simulink model "dentrosis"  (R2024b)
settings: Solver=ode45  StartTime=0.0  StopTime=10.0  MaxStep=1e-3  RelTol=1e-3
libraries: slpidlib x1
settings Model: Creator=Dell
settings DataIOCC: ReturnWorkspaceOutputs=off  TimeSaveName=t
settings DebuggingCC: AlgebraicLoopMsg=none  ArtificialAlgebraicLoopMsg=none  InheritedTsInSrcMsg=none
settings RTWCC: GPUComputeCapability=3.5

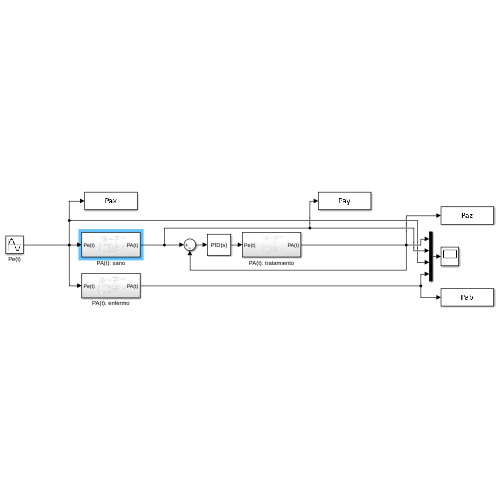
[thumbnail: Simulink's stored preview of the top-level diagram]
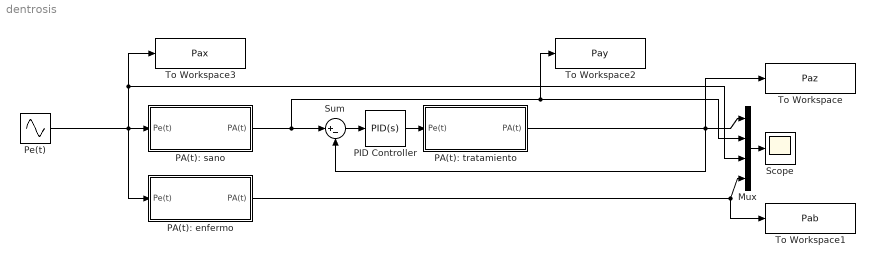
== system dentrosis ==
  Mux : Mux
  PA(t): enfermo : Subsystem
  PA(t): sano : Subsystem
  PA(t): tratamiento : Subsystem
  PID Controller : slpidlib/PID Controller  Controller=PID  Form=Parallel  TimeDomain=Continuous-time  UseExternalTs=off  SampleTime=-1  IntegratorMethod=Forward Euler  FilterMethod=Forward Euler  ControllerParametersSource=internal  P=7504.3128  I=40028.7836  UseKiTs=off  D=312.5866  UseExternalDerivativeSource=off  N=104491.5556  UseFilter=on  TunerSelectOption=Transfer Function Based (PID Tuner App)  InitialConditionSource=internal  InitialConditionForIntegrator=0  InitialConditionForFilter=0  DifferentiatorICPrevScaledInput=0  ExternalReset=none  TrackingMode=off  Kt=1  LimitOutput=off  SatLimitsSource=internal  UpperSaturationLimit=inf  LowerSaturationLimit=-inf  LinearizeAsGain=on  AntiWindupMode=none  Kb=1  LimitIntegrator=off  UpperIntegratorSaturationLimit=inf  LowerIntegratorSaturationLimit=-inf  POutMin=[]  POutMax=[]  IOutMin=[]  IOutMax=[]  DOutMin=[]  DOutMax=[]  NOutMin=[]  NOutMax=[]  SumOutMin=[]  SumOutMax=[]  SaturationOutMin=[]  SaturationOutMax=[]  PParamMin=[]  PParamMax=[]  IParamMin=[]  IParamMax=[]  DParamMin=[]  DParamMax=[]  NParamMin=[]  NParamMax=[]  KbParamMin=[]  KbParamMax=[]  KtParamMin=[]  KtParamMax=[]  KbOutMin=[]  KbOutMax=[]  KtOutMin=[]  KtOutMax=[]  IntegratorOutMin=[]  IntegratorOutMax=[]  FilterOutMin=[]  FilterOutMax=[]  SumI1OutMin=[]  SumI1OutMax=[]  SumI2OutMin=[]  SumI2OutMax=[]  SumI3OutMin=[]  SumI3OutMax=[]  SumI4OutMin=[]  SumI4OutMax=[]  SumDOutMin=[]  SumDOutMax=[]  DifferentiatorOutMin=[]  DifferentiatorOutMax=[]  FilterDiffOutCoefMin=[]  FilterDiffOutCoefMax=[]  ReciprocalOutMin=[]  ReciprocalOutMax=[]  SumDenOutMin=[]  SumDenOutMax=[]  SumNumOutMin=[]  SumNumOutMax=[]  DivideOutMin=[]  DivideOutMax=[]  UdiffTsProdOutMin=[]  UdiffTsProdOutMax=[]  NTsProdOutMin=[]  NTsProdOutMax=[]  UintegralTsProdOutMin=[]  UintegralTsProdOutMax=[]  UngainTsProdOutMin=[]  UngainTsProdOutMax=[]  ClampingZeroOutDataTypeStr=Inherit: Inherit via back propagation  ClampingZeroOutMin=[]  ClampingZeroOutMax=[]  FilterDenConstantOutDataTypeStr=Inherit: Inherit via back propagation  FilterDenConstantOutMin=[]  FilterDenConstantOutMax=[]  PCopyOutDataTypeStr=Inherit: Inherit via back propagation  PCopyOutMin=[]  PCopyOutMax=[]  NCopyOutDataTypeStr=Inherit: Inherit via back propagation  NCopyOutMin=[]  NCopyOutMax=[]  IntegratorContinuousStateAttributes=''  IntegratorStateMustResolveToSignalObject=off  IntegratorRTWStateStorageClass=Auto  FilterContinuousStateAttributes=''  FilterStateMustResolveToSignalObject=off  FilterRTWStateStorageClass=Auto  ParallelPVariant=InternalParameters  IdealPVariant=Disabled  IVariant=InternalParameters  DVariant=InternalParameters  IntegratorVariant=Continuous  SatVariant=Disabled  AWVariant=Passthrough  PCopyVariant=Disabled  TRVariant=Disabled  FdbkBlocksVariant=Forward  IdealPFdbkVariant=Disabled  SatFdbkVariant=Disabled  DerivativeFilterVariant=ContFilter  NVariant=InternalParameters  NCopyVariant=Disabled  FilterICVariant=InternalICsFilter  IntegratorICVariant=InternalICs  ExternalResetVariant=Disabled  TRSumVariant=Passthrough  SumFdbkVariant=Disabled  SumVariant=Sum_PID  TsampFilterVariant=InternalTs  TsampNgainVariant=Passthrough  TsampIntegralVariant=Disabled_SignalSpec  ExternalSaturationOutDataTypeStr=Inherit: Same as second input  DerivativeSourceVariant=ErrorSignal  PreIntVariant=InternalPreInt
  Pe(t) : Sin  Frequency=1.5
  Scope : Scope
  Sum : Sum  Inputs=|+-
  To Workspace : ToWorkspace  VariableName=Paz  SampleTime=-1
  To Workspace1 : ToWorkspace  VariableName=Pab  SampleTime=-1
  To Workspace2 : ToWorkspace  VariableName=Pay  SampleTime=-1
  To Workspace3 : ToWorkspace  VariableName=Pax  SampleTime=-1
  wires:
  Mux/1 -> Scope/1
  Sum/1 -> PID Controller/1
  PID Controller/1 -> PA(t): tratamiento/1(Pe(t))
  PA(t): tratamiento/1(PA(t)) -> To Workspace/1, Mux/1, Sum/2
  PA(t): sano/1(PA(t)) -> To Workspace2/1, Mux/2, Sum/1
  Pe(t)/1 -> PA(t): enfermo/1(Pe(t)), PA(t): sano/1(Pe(t)), To Workspace3/1, Mux/3
  PA(t): enfermo/1(PA(t)) -> To Workspace1/1, Mux/4

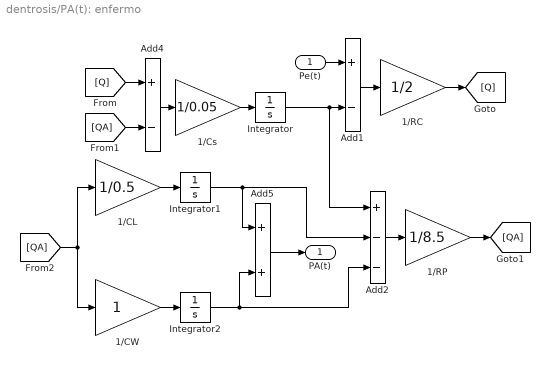
== system dentrosis/PA(t): enfermo ==
  Pe(t) : Inport
  1/CL : Gain  Gain=1/0.5
  1/CW : Gain
  1/Cs : Gain  Gain=1/0.05
  1/RC : Gain  Gain=1/2
  1/RP : Gain  Gain=1/8.5
  Add1 : Sum  Inputs=+-
  Add2 : Sum  Inputs=+--
  Add4 : Sum  Inputs=+-
  Add5 : Sum
  Integrator : Integrator
  Integrator1 : Integrator
  Integrator2 : Integrator
  PA(t) : Outport
  wires:
  1/RC/1 -> [Q]
  Add1/1 -> 1/RC/1
  1/RP/1 -> [QA]
  Add2/1 -> 1/RP/1
  [Q] -> Add4/1
  [QA] -> Add4/2
  Add4/1 -> 1/Cs/1
  1/Cs/1 -> Integrator/1
  Pe(t)/1 -> Add1/1
  [QA] -> 1/CL/1, 1/CW/1
  1/CL/1 -> Integrator1/1
  1/CW/1 -> Integrator2/1
  Add5/1 -> PA(t)/1
  Integrator2/1 -> Add5/2, Add2/3
  Integrator/1 -> Add2/1, Add1/2
  Integrator1/1 -> Add5/1, Add2/2

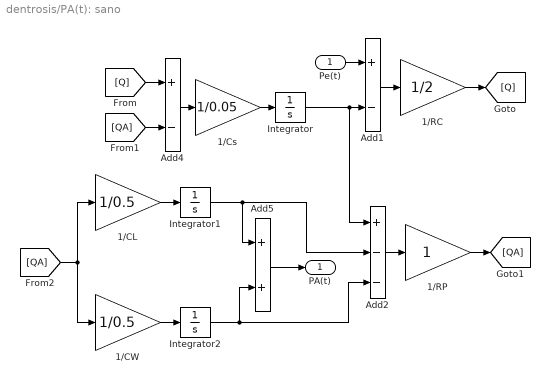
== system dentrosis/PA(t): sano ==
  Pe(t) : Inport
  1/CL : Gain  Gain=1/0.5
  1/CW : Gain  Gain=1/0.5
  1/Cs : Gain  Gain=1/0.05
  1/RC : Gain  Gain=1/2
  1/RP : Gain
  Add1 : Sum  Inputs=+-
  Add2 : Sum  Inputs=+--
  Add4 : Sum  Inputs=+-
  Add5 : Sum
  Integrator : Integrator
  Integrator1 : Integrator
  Integrator2 : Integrator
  PA(t) : Outport
  wires:
  1/RC/1 -> [Q]
  Add1/1 -> 1/RC/1
  1/RP/1 -> [QA]
  Add2/1 -> 1/RP/1
  [Q] -> Add4/1
  [QA] -> Add4/2
  Add4/1 -> 1/Cs/1
  1/Cs/1 -> Integrator/1
  Pe(t)/1 -> Add1/1
  [QA] -> 1/CL/1, 1/CW/1
  1/CL/1 -> Integrator1/1
  1/CW/1 -> Integrator2/1
  Add5/1 -> PA(t)/1
  Integrator2/1 -> Add5/2, Add2/3
  Integrator/1 -> Add2/1, Add1/2
  Integrator1/1 -> Add5/1, Add2/2

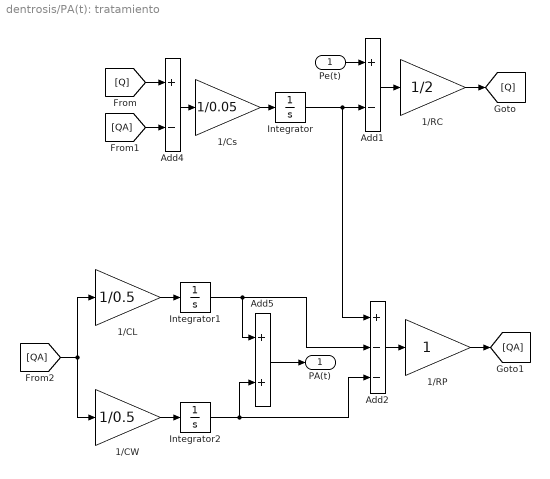
== system dentrosis/PA(t): tratamiento ==
  Pe(t) : Inport
  1/CL : Gain  Gain=1/0.5
  1/CW : Gain  Gain=1/0.5
  1/Cs : Gain  Gain=1/0.05
  1/RC : Gain  Gain=1/2
  1/RP : Gain
  Add1 : Sum  Inputs=+-
  Add2 : Sum  Inputs=+--
  Add4 : Sum  Inputs=+-
  Add5 : Sum
  Integrator : Integrator
  Integrator1 : Integrator
  Integrator2 : Integrator
  PA(t) : Outport
  wires:
  1/RC/1 -> [Q]
  Add1/1 -> 1/RC/1
  1/RP/1 -> [QA]
  Add2/1 -> 1/RP/1
  [Q] -> Add4/1
  [QA] -> Add4/2
  Add4/1 -> 1/Cs/1
  1/Cs/1 -> Integrator/1
  Pe(t)/1 -> Add1/1
  [QA] -> 1/CL/1, 1/CW/1
  1/CL/1 -> Integrator1/1
  1/CW/1 -> Integrator2/1
  Add5/1 -> PA(t)/1
  Integrator2/1 -> Add5/2, Add2/3
  Integrator/1 -> Add2/1, Add1/2
  Integrator1/1 -> Add5/1, Add2/2
